simulink model "task7_lab13"  (R2021a)
settings: Solver=VariableStepAuto  StartTime=0.0  StopTime=10.0  RelTol=1e-3
settings Model: Creator=reemb  LastModifiedBy=reemb

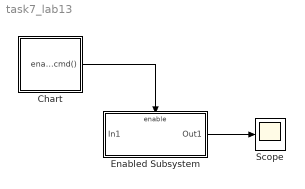
== system task7_lab13 ==
  Chart : Stateflow chart  TreatAsAtomicUnit=on
  Enabled Subsystem : Subsystem  TreatAsAtomicUnit=on
  Scope : Scope
  wires:
  Enabled Subsystem/1(Out1) -> Scope/1
  Chart/1(enable_cmd()) -> Enabled Subsystem/Enable

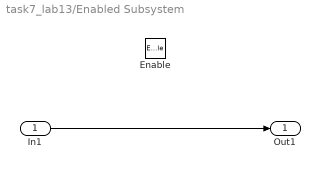
== system task7_lab13/Enabled Subsystem ==
  In1 : Inport
  Enable : EnablePort
  Out1 : Outport
  wires:
  In1/1 -> Out1/1

== stateflow chart task7_lab13/Chart ==
  state a
    during: enable_cmd;
  state a1
  a1 -> a : after(3, sec)
  (default) -> a
  a -> a1 : after(3, sec)
  events: enable_cmd output FUNCTION_CALL_EVENT
